simulink model "Lab2_1"  (R2012b)
settings: Solver=ode45  StartTime=0.0  StopTime=100  RelTol=1e-3
libraries: simulink_extras x2, simulink x1
settings Model: Creator=Viktor  LastModifiedBy=Viktor

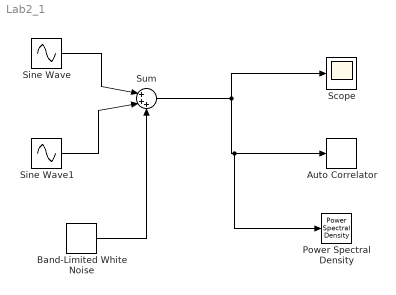
== system Lab2_1 ==
  Auto Correlator : simulink_extras/Additional Sinks/Auto Correlator  npts=100  HowOften=50  sampleT=0.1
  Band-Limited White Noise : simulink/Sources/Band-Limited White Noise  Cov=[1]  Ts=0.1  seed=[23341]
  Power Spectral Density : simulink_extras/Additional Sinks/Power Spectral Density  npts=128  fftpts=512  HowOften=64  sampleT=0.1
  Scope : Scope
  Sine Wave : Sin  Frequency=10  SampleTime=0
  Sine Wave1 : Sin  Frequency=5  SampleTime=0
  Sum : Sum  Inputs=|+++
  wires:
  Sum/1 -> Scope/1, Power Spectral Density/1, Auto Correlator/1
  Band-Limited White Noise/1 -> Sum/3
  Sine Wave1/1 -> Sum/2
  Sine Wave/1 -> Sum/1
